simulink library "lib_mod_operation"  (R2023a)
settings: Solver=VariableStepAuto  StartTime=0.0  StopTime=10.0  RelTol=1e-3
libraries: lib_conversion x1
settings Model: Creator=cav2ofo  LastModifiedBy=lenovo
settings OptimizationCC: ReuseModelBlockBuffer=off

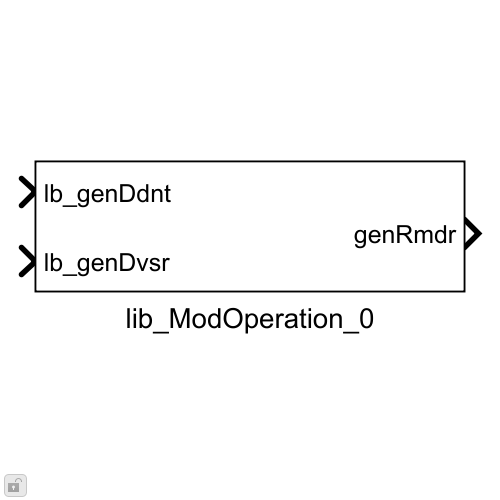
[thumbnail: Simulink's stored preview of the top-level diagram]
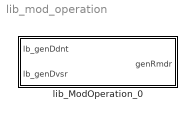
== system lib_mod_operation ==
  lib_ModOperation_0 : Subsystem  mask{lb_parOutpDataType=Inherit: Inherit via back propagation}
      mask prompts: lb_parOutpDataType "Output Datatype:"
      mask DialogControl DescGroupVar Prompt: Modulo block
      mask DialogControl DescTextVar Prompt: This block is a custom implmentation of MOD/modulo operation. It output remainder by when an input number (Divident) is divided by anothor number (Divisor).
      mask DialogControl ParameterGroupVar Prompt: Output Parameter

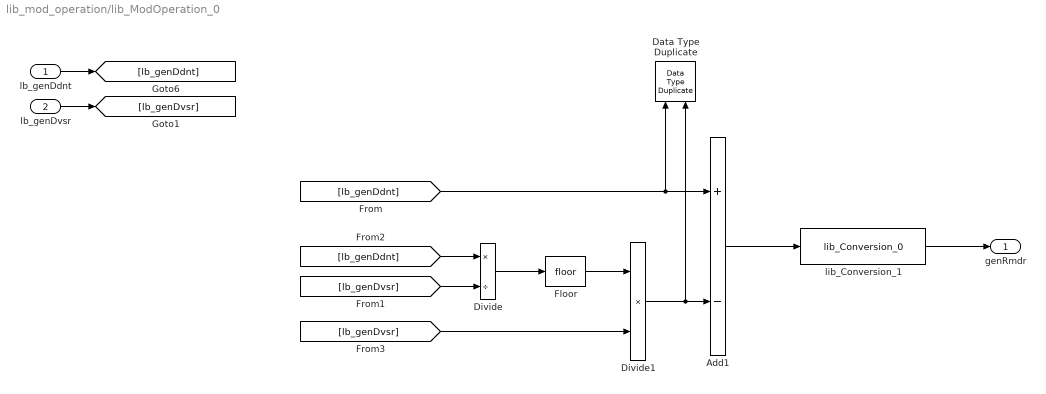
== system lib_mod_operation/lib_ModOperation_0 ==
  lb_genDdnt : Inport
  lb_genDvsr : Inport  Port=2
  Add1 : Sum  Inputs=+-  OutDataTypeStr=Inherit: Inherit via back propagation
  Data Type Duplicate : DataTypeDuplicate
  Divide : Product  Inputs=*/  OutDataTypeStr=single
  Divide1 : Product  Inputs=**  OutDataTypeStr=Inherit: Inherit via back propagation
  Floor : Rounding
  lib_Conversion_1 : lib_conversion/lib_Conversion_0  lb_parDataType=lb_parOutpDataType  lb_parOutpMaxVal=[]  lb_parOutpMinVal=[]  lb_parSatFlag=off
  genRmdr : Outport
  wires:
  [lb_genDvsr] -> Divide/2
  Add1/1 -> lib_Conversion_1/1
  Floor/1 -> Divide1/1
  Divide/1 -> Floor/1
  [lb_genDdnt] -> Data Type Duplicate/1, Add1/1
  lb_genDdnt/1 -> [lb_genDdnt]
  lb_genDvsr/1 -> [lb_genDvsr]
  [lb_genDdnt] -> Divide/1
  [lb_genDvsr] -> Divide1/2
  lib_Conversion_1/1 -> genRmdr/1
  Divide1/1 -> Data Type Duplicate/2, Add1/2
